simulink model "flightgear_simulator"  (R2019b)
settings: Solver=VariableStepAuto  StartTime=0.0  StopTime=simt  RelTol=1e-3
values from neighbouring files (symbols this model uses):
  dt = simout.t(2)-simout.t(1)    [main.m]
  originlat = 64.650532    [main.m]
  originlon = -147.066893    [main.m]
undefined symbols (not defined in the file or in its folder): Earth, WGS84
libraries: aerolibtransform2 x1, aerolibfltsims x1
settings Model: Creator=Usuario  LastModifiedBy=Usuario

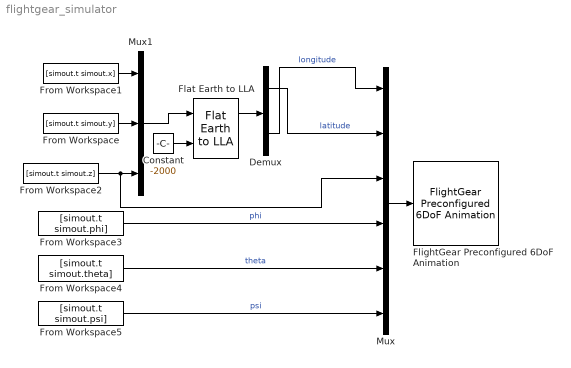
== system flightgear_simulator ==
  Constant : Constant  Value=-2000  SampleTime=dt
  Demux : Demux  Outputs=2
  Flat Earth to LLA : aerolibtransform2/Flat Earth to LLA  units=Metric (MKS)  ptype=Earth (WGS84)  F=1/298.257223563  R=6378137  LL0=[originlat originlon]  psi=0
  FlightGear Preconfigured 6DoF Animation : aerolibfltsims/FlightGear Preconfigured 6DoF Animation  xFlightGearVersion=v2018.3  DestinationIpAddress=127.0.0.1  DestinationPort=5502  SampleTime=dt  packetVersion=24
      settings: SourceProductName=Aerospace Blockset
  From Workspace : FromWorkspace  VariableName=[simout.t simout.y]  SampleTime=dt
  From Workspace1 : FromWorkspace  VariableName=[simout.t simout.x]  SampleTime=dt
  From Workspace2 : FromWorkspace  VariableName=[simout.t simout.z]  SampleTime=dt
  From Workspace3 : FromWorkspace  VariableName=[simout.t simout.phi]  SampleTime=dt
  From Workspace4 : FromWorkspace  VariableName=[simout.t simout.theta]  SampleTime=dt
  From Workspace5 : FromWorkspace  VariableName=[simout.t simout.psi]  SampleTime=dt
  Mux : Mux  Inputs=6
  Mux1 : Mux  Inputs=3
  wires:
  Mux/1 -> FlightGear Preconfigured 6DoF Animation/1
  Constant/1 -> Flat Earth to LLA/2
  Flat Earth to LLA/1 -> Demux/1
  From Workspace5/1 -> Mux/6  "psi"
  From Workspace4/1 -> Mux/5  "theta"
  From Workspace3/1 -> Mux/4  "phi"
  Demux/1 -> Mux/2  "latitude"
  Demux/2 -> Mux/1  "longitude"
  Mux1/1 -> Flat Earth to LLA/1
  From Workspace/1 -> Mux1/2
  From Workspace1/1 -> Mux1/1
  From Workspace2/1 -> Mux/3, Mux1/3
